simulink model "PID_fuzzy_app"  (Simulink 7.8)
settings: Solver=ode3  StartTime=0.0  StopTime=10  FixedStep=0.01  RelTol=1e-3
libraries: fuzblock x3
settings Model: Creator=a2791ft  LastModifiedBy=Cohen
settings SolverCC: MaxConsecutiveZCs=1e6  ZeroCrossControl=DisableAll
settings OptimizationCC: InitFltsAndDblsToZero=on
settings DebuggingCC: FcnCallInpInsideContextMsg=Use local settings  StrictBusMsg=Warning

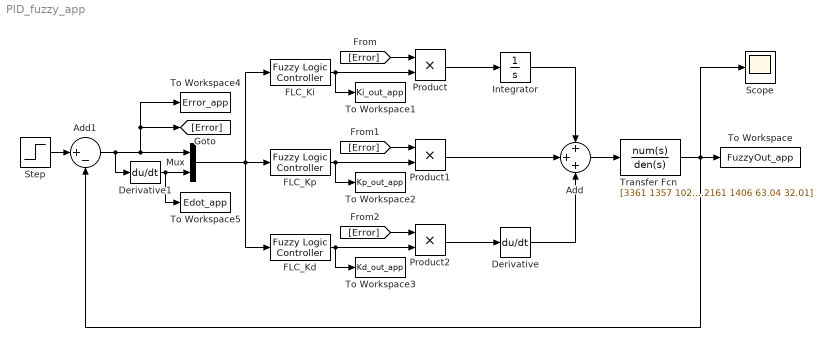
== system PID_fuzzy_app ==
  Add : Sum  Inputs=+++
  Add1 : Sum  Inputs=|+-
  Derivative : Derivative  CoefficientInTFapproximation=-1
  Derivative1 : Derivative
  FLC_Kd : fuzblock/Fuzzy Logic  Controller  fis=Kdfz
  FLC_Ki : fuzblock/Fuzzy Logic  Controller  fis=Kifz
  FLC_Kp : fuzblock/Fuzzy Logic  Controller  fis=Kpfz
  Integrator : Integrator
  Mux : Mux  Inputs=2
  Product : Product  RndMeth=Zero
  Product1 : Product  RndMeth=Zero
  Product2 : Product  RndMeth=Zero
  Scope : Scope
  Step : Step  SampleTime=0
  To Workspace : ToWorkspace  VariableName=FuzzyOut_app  SampleTime=-1  SaveFormat=Structure With Time
  To Workspace1 : ToWorkspace  VariableName=Ki_out_app  SampleTime=-1  SaveFormat=Structure With Time
  To Workspace2 : ToWorkspace  VariableName=Kp_out_app  SampleTime=-1  SaveFormat=Structure With Time
  To Workspace3 : ToWorkspace  VariableName=Kd_out_app  SampleTime=-1  SaveFormat=Structure With Time
  To Workspace4 : ToWorkspace  VariableName=Error_app  SampleTime=-1  SaveFormat=Structure With Time
  To Workspace5 : ToWorkspace  VariableName=Edot_app  SampleTime=-1  SaveFormat=Structure With Time
  Transfer Fcn : TransferFcn  Numerator=[3361 1357 102.2]  Denominator=[230.6 2508 2161 1406 63.04 32.01]
  wires:
  Step/1 -> Add1/1
  Transfer Fcn/1 -> To Workspace/1, Add1/2, Scope/1
  Add/1 -> Transfer Fcn/1
  Mux/1 -> FLC_Kp/1, FLC_Ki/1, FLC_Kd/1
  Integrator/1 -> Add/1
  Derivative/1 -> Add/3
  Add1/1 -> Derivative1/1, Mux/1, [Error], To Workspace4/1
  Derivative1/1 -> Mux/2, To Workspace5/1
  Product/1 -> Integrator/1
  FLC_Ki/1 -> Product/2, To Workspace1/1
  Product1/1 -> Add/2
  FLC_Kp/1 -> Product1/2, To Workspace2/1
  Product2/1 -> Derivative/1
  FLC_Kd/1 -> Product2/2, To Workspace3/1
  [Error] -> Product/1
  [Error] -> Product1/1
  [Error] -> Product2/1
